simulink model "lane_detection_model"  (R2026a)
settings: Solver=VariableStepAuto
settings Model: Creator=svvb7  LastModifiedBy=svvb7

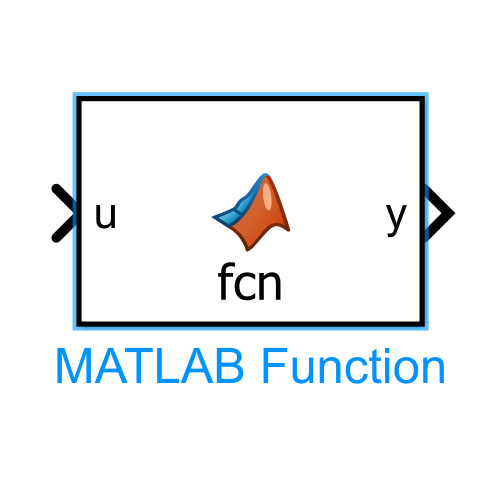
[thumbnail: Simulink's stored preview of the top-level diagram]
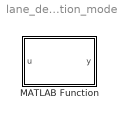
== system lane_detection_model ==
  MATLAB Function : MATLAB Function  TreatAsAtomicUnit=on

== matlab function lane_detection_model/MATLAB Function ==
  data: u input; y output
function y = fcn(u)
clc;
clear;
close all;

model = 'lane_detection_model';

new_system(model);

open_system(model);

% Add blocks
add_block('simulink/Sources/In1', ...
    [model '/Image_Input']);

add_block('simulink/Math Operations/Gain', ...
    [model '/Gray_Conversion']);

add_block('simulink/Discrete/Discrete Filter', ...
    [model '/Gaussian_Filter']);

add_block('simulink/Math Operations/Add', ...
    [model '/Edge_Detection']);

add_block('simulink/Sinks/Out1', ...
    [model '/Lane_Output']);

% Connect blocks
add_line(model,'Image_Input/1','Gray_Conversion/1');

add_line(model,'Gray_Conversion/1','Gaussian_Filter/1');

add_line(model,'Gaussian_Filter/1','Edge_Detection/1');

add_line(model,'Edge_Detection/1','Lane_Output/1');

save_system(model);

open_system(model);
